simulink model "pendulo_dmc"  (Simulink 7.9)
settings: Solver=ode45  StartTime=0.0  StopTime=20  FixedStep=T  RelTol=1e-3
undefined symbols (not defined in the file or in its folder): b, g, grav, L, m, T, yp_equilibrio
settings Model: Creator=Kawakami  LastModifiedBy=Kawakami
settings DataIOCC: SignalLoggingName=sigsOut
settings OptimizationCC: BooleanDataType=off
settings DebuggingCC: SaveWithParameterizedLinksMsg=none  SignalResolutionControl=TryResolveAllWithWarning  SolverPrmCheckMsg=none  MultiTaskDSMMsg=warning  MultiTaskCondExecSysMsg=none  FcnCallInpInsideContextMsg=Use local settings  StrictBusMsg=None
settings HardwareCC: TargetUnknown=on
settings RTWCC: IncludeERTFirstTime=on
settings GRTTargetCC: CombineOutputUpdateFcns=off  GRTInterface=on

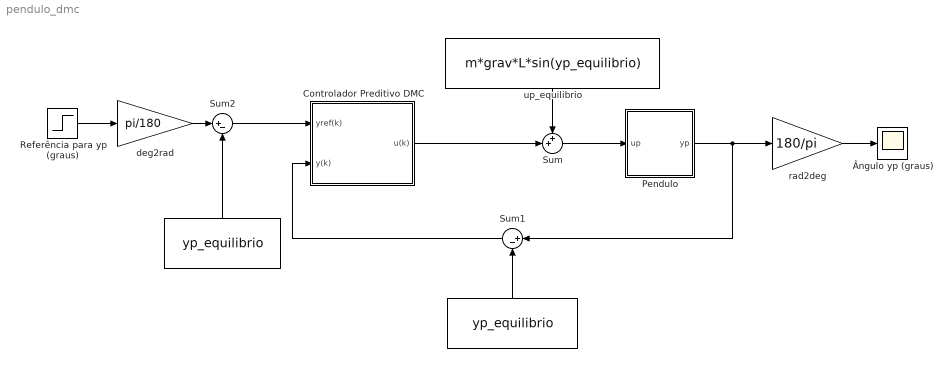
== system pendulo_dmc ==
  " " : Constant  Value=yp_equilibrio
  "  " : Constant  Value=yp_equilibrio
  Controlador Preditivo DMC : Subsystem  mask{rho=0.3, N=50, M=10, g=g, T=T}
      mask prompts: rho "Peso do controle (rho)"; N "Horizonte de Predição (N)"; M "Horizonte de Controle (M)"; g "Resposta a degrau da planta (g)"; T "Período de amostragem (T)"
      mask init:
      | Ns = length(g);
      | gaux = g;
      | if N > Ns
      |     gaux(Ns+1:N) = g(Ns);
      | end
      | col = gaux(1:N);
      | row = [gaux(1) zeros(1,N-1)];
      | G = toeplitz(col,row);
      | G = G(:,1:M);
      | GAIN = inv(G'*G + rho*eye(M))*G';
      | KDMC = GAIN(1,:);
  Pendulo : Subsystem  mask{m=m, L=L, grav=grav, b=b, theta0=yp_equilibrio}
      mask prompts: m "m (kg)"; L "L (m)"; grav "grav (m/s^2)"; b "b (Ns/(m*rad))"; theta0 "theta inicial (rad)"
  Referência para yp (graus) : Step  Time=10  Before=yp_equilibrio*180/pi  After=(yp_equilibrio*180/pi) + 10  SampleTime=0
  Sum : Sum  Inputs=++|  SaturateOnIntegerOverflow=on
  Sum1 : Sum  Inputs=|+-  SaturateOnIntegerOverflow=on
  Sum2 : Sum  Inputs=|+-  SaturateOnIntegerOverflow=on
  deg2rad : Gain  Gain=pi/180  SaturateOnIntegerOverflow=on  OutDataTypeStr=Inherit: Same as input  ParamDataTypeStr=Inherit: Same as input
  rad2deg : Gain  Gain=180/pi  SaturateOnIntegerOverflow=on  OutDataTypeStr=Inherit: Same as input  ParamDataTypeStr=Inherit: Same as input
  up_equilibrio : Constant  Value=m*grav*L*sin(yp_equilibrio)
  Ângulo yp (graus) : Scope
      settings: TimeRange=20  YMin=58  YMax=72  SaveName=y
  wires:
  Pendulo/1(yp) -> Sum1/1, rad2deg/1
  Controlador Preditivo DMC/1(u(k)) -> Sum/2
  Sum/1 -> Pendulo/1(up)
  Sum1/1 -> Controlador Preditivo DMC/2(y(k))
  Sum2/1 -> Controlador Preditivo DMC/1(yref(k))
  Referência para yp (graus)/1 -> deg2rad/1
  deg2rad/1 -> Sum2/1
  rad2deg/1 -> Ângulo yp (graus)/1
  up_equilibrio/1 -> Sum/1
  "  "/1 -> Sum2/2
  " "/1 -> Sum1/2

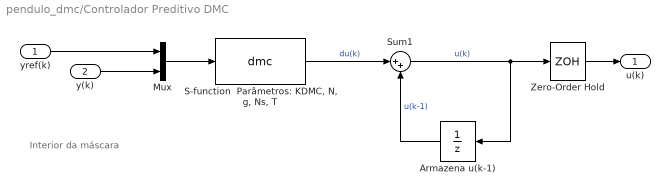
== system pendulo_dmc/Controlador Preditivo DMC ==
  note: Interior da
      | máscara
  yref(k) : Inport
  y(k) : Inport  Port=2
  Armazena u(k-1) : UnitDelay  SampleTime=T
  Mux : Mux  Inputs=2
  "S-function  Parâmetros: KDMC, N, g, Ns, T" : S-Function  FunctionName=dmc  Parameters=KDMC,N,g,Ns,T  EnableBusSupport=off
  Sum1 : Sum  Inputs=|++  SaturateOnIntegerOverflow=on  InputSameDT=on  OutDataTypeStr=Inherit: Same as first input
  Zero-Order Hold : ZeroOrderHold  SampleTime=T
  u(k) : Outport
  wires:
  Mux/1 -> "S-function  Parâmetros: KDMC, N, g, Ns, T"/1
  Zero-Order Hold/1 -> u(k)/1
  y(k)/1 -> Mux/2
  yref(k)/1 -> Mux/1
  Sum1/1 -> Zero-Order Hold/1, Armazena u(k-1)/1  "u(k)"
  Armazena u(k-1)/1 -> Sum1/2  "u(k-1)"
  "S-function  Parâmetros: KDMC, N, g, Ns, T"/1 -> Sum1/1  "du(k)"

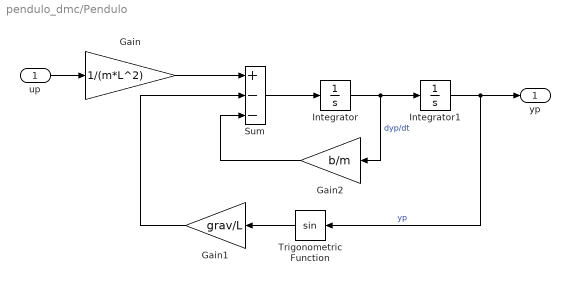
== system pendulo_dmc/Pendulo ==
  up : Inport
  Gain : Gain  Gain=1/(m*L^2)  SaturateOnIntegerOverflow=on  OutDataTypeStr=Inherit: Same as input  ParamDataTypeStr=Inherit: Same as input
  Gain1 : Gain  Gain=grav/L  SaturateOnIntegerOverflow=on  OutDataTypeStr=Inherit: Same as input  ParamDataTypeStr=Inherit: Same as input
  Gain2 : Gain  Gain=b/m  SaturateOnIntegerOverflow=on  OutDataTypeStr=Inherit: Same as input  ParamDataTypeStr=Inherit: Same as input
  Integrator : Integrator
  Integrator1 : Integrator  InitialCondition=theta0
  Sum : Sum  Inputs=+--  SaturateOnIntegerOverflow=on
  Trigonometric Function : Trigonometry
  yp : Outport
  wires:
  Integrator/1 -> Integrator1/1, Gain2/1  "dyp/dt"
  Sum/1 -> Integrator/1
  Gain/1 -> Sum/1
  Trigonometric Function/1 -> Gain1/1
  Integrator1/1 -> Trigonometric Function/1, yp/1  "yp"
  Gain1/1 -> Sum/2
  Gain2/1 -> Sum/3
  up/1 -> Gain/1
